simulink model "Cathode_Simscape_Model"  (R2023a)
settings: Solver=VariableStepAuto  StartTime=0.0  StopTime=500  RelTol=1e-3
settings Model: Creator=mahesh.kumar  LastModifiedBy=mahesh.kumar

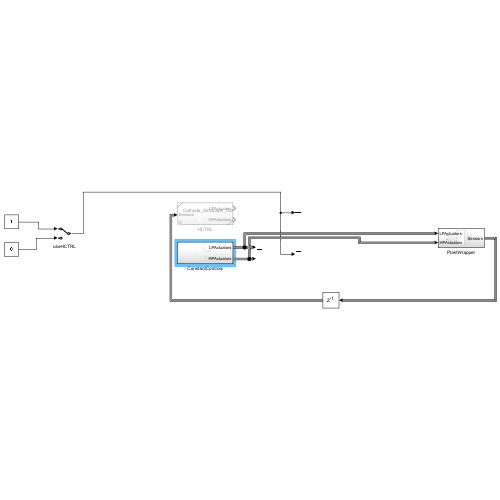
[thumbnail: Simulink's stored preview of the top-level diagram]
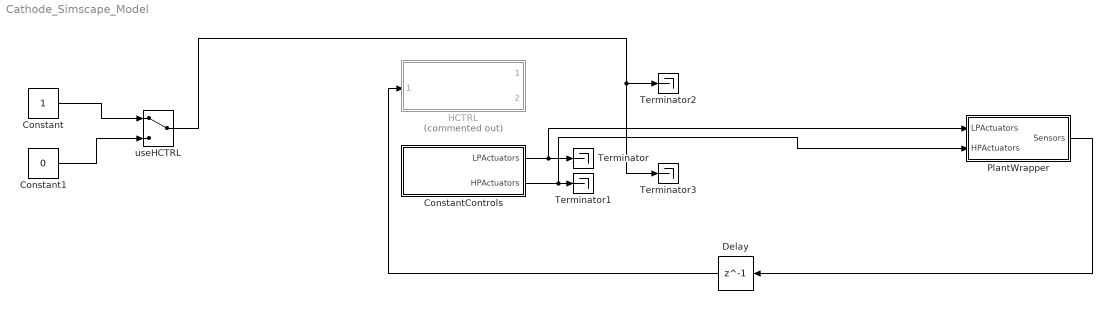
== system Cathode_Simscape_Model ==
  Constant : Constant  OutDataTypeStr=boolean
  Constant1 : Constant  Value=0  OutDataTypeStr=boolean
  ConstantControls : Subsystem
  Delay : Delay  DelayLength=1
  HCTRL : Subsystem  Commented=on  ReferencedSubsystem=Cathode_Simscape_ControllerWrapper_RefSub
  PlantWrapper : Subsystem
  Terminator{,1..3} (4 alike) : Terminator
  useHCTRL : ManualSwitch
  wires:
  Constant/1 -> useHCTRL/1
  Constant1/1 -> useHCTRL/2
  useHCTRL/1 -> Terminator3/1, Terminator2/1
  PlantWrapper/1(Sensors) -> Delay/1
  Delay/1 -> HCTRL/1
  ConstantControls/1(LPActuators) -> PlantWrapper/1(LPActuators), Terminator/1
  ConstantControls/2(HPActuators) -> PlantWrapper/2(HPActuators), Terminator1/1

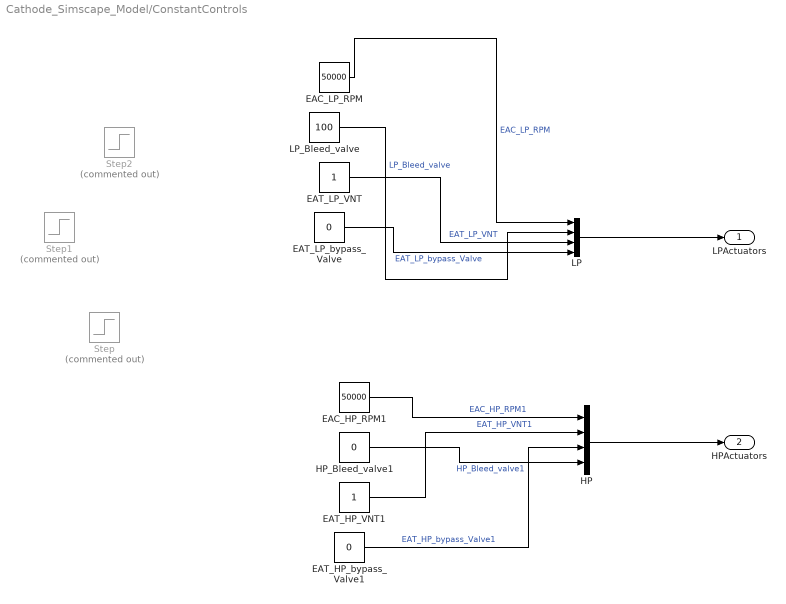
== system Cathode_Simscape_Model/ConstantControls ==
  EAC_HP_RPM1 : Constant  Value=50000
  EAC_LP_RPM : Constant  Value=50000
  EAT_HP_VNT1 : Constant
  EAT_HP_bypass_Valve1 : Constant  Value=0
  EAT_LP_VNT : Constant
  EAT_LP_bypass_Valve : Constant  Value=0
  HP : BusCreator  Inputs=4
  HP_Bleed_valve1 : Constant  Value=0
  LP : BusCreator  Inputs=4
  LP_Bleed_valve : Constant  Value=100
  Step : Step  Commented=on  Time=250  Before=50000  After=60000  SampleTime=0
  Step1 : Step  Commented=on  Time=250  Before=50000  After=60000  SampleTime=0
  Step2 : Step  Commented=on  Time=250  After=50  SampleTime=0
  LPActuators : Outport
  HPActuators : Outport  Port=2
  wires:
  EAT_HP_bypass_Valve1/1 -> HP/3  "EAT_HP_bypass_Valve1"
  EAT_LP_bypass_Valve/1 -> LP/4  "EAT_LP_bypass_Valve"
  EAC_HP_RPM1/1 -> HP/1  "EAC_HP_RPM1"
  EAT_LP_VNT/1 -> LP/3  "EAT_LP_VNT"
  HP_Bleed_valve1/1 -> HP/4  "HP_Bleed_valve1"
  LP_Bleed_valve/1 -> LP/2  "LP_Bleed_valve"
  EAT_HP_VNT1/1 -> HP/2  "EAT_HP_VNT1"
  LP/1 -> LPActuators/1
  HP/1 -> HPActuators/1
  EAC_LP_RPM/1 -> LP/1  "EAC_LP_RPM"

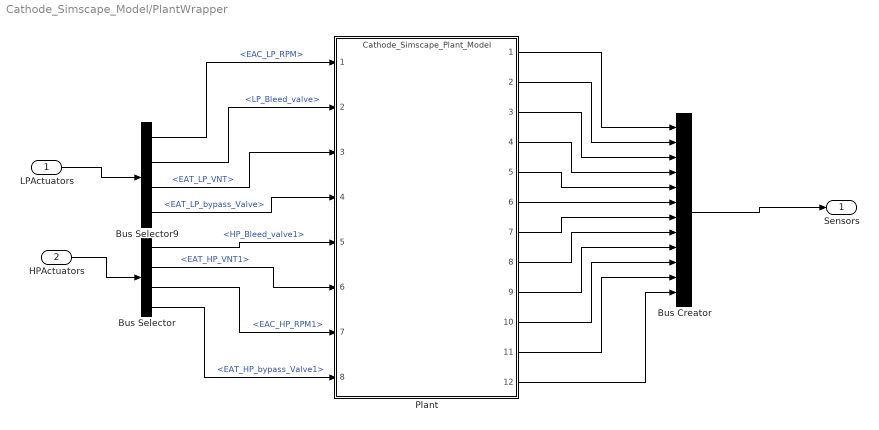
== system Cathode_Simscape_Model/PlantWrapper ==
  LPActuators : Inport
  HPActuators : Inport  Port=2
  Bus Creator : BusCreator  Inputs=12
  Bus Selector : BusSelector  OutputSignals=HP_Bleed_valve1,EAT_HP_VNT1,EAC_HP_RPM1,EAT_HP_bypass_Valve1
  Bus Selector9 : BusSelector  OutputSignals=EAC_LP_RPM,LP_Bleed_valve,EAT_LP_VNT,EAT_LP_bypass_Valve
  Plant : ModelReference  ModelNameDialog=Cathode_Simscape_Plant_Model  SimulationMode=Normal  ModelReferenceVersion=1.23
  Sensors : Outport
  wires:
  Plant/6 -> Bus Creator/6
  Plant/5 -> Bus Creator/5
  Bus Selector/4 -> Plant/8  "<EAT_HP_bypass_Valve1>"
  Bus Selector9/4 -> Plant/4  "<EAT_LP_bypass_Valve>"
  Plant/11 -> Bus Creator/11
  Plant/4 -> Bus Creator/4
  Plant/7 -> Bus Creator/7
  Bus Selector9/3 -> Plant/3  "<EAT_LP_VNT>"
  Plant/1 -> Bus Creator/1
  Plant/2 -> Bus Creator/2
  Bus Selector9/2 -> Plant/2  "<LP_Bleed_valve>"
  Bus Creator/1 -> Sensors/1
  Bus Selector/2 -> Plant/6  "<EAT_HP_VNT1>"
  Bus Selector9/1 -> Plant/1  "<EAC_LP_RPM>"
  Plant/8 -> Bus Creator/8
  Plant/3 -> Bus Creator/3
  Bus Selector/3 -> Plant/7  "<EAC_HP_RPM1>"
  Plant/10 -> Bus Creator/10
  Bus Selector/1 -> Plant/5  "<HP_Bleed_valve1>"
  Plant/9 -> Bus Creator/9
  HPActuators/1 -> Bus Selector/1
  LPActuators/1 -> Bus Selector9/1
  Plant/12 -> Bus Creator/12
